simulink model "DA40_Flight_Model"  (R2023a)
settings: Solver=FixedStepAuto  StartTime=Start_Time  StopTime=End_Time  FixedStep=Time_Step  RelTol=1e-3
values from neighbouring files (symbols this model uses):
  BSFC_LUT = aircraft.BSFC_LUT    [NavigationProcessor.m]    (also in ReceiverPositions.m = obj.aircraft.BSFC_LUT; VectorTracking.m = load("DA40ENGINE.mat"))
  clkVar = formClkVariance(aircraft.clockType,1/aircraft.frequency)    [initializeSim.m]
  initP = blkdiag(diag([0.1 0.1 0.1]),diag([pi/90 pi/90 pi/90]),diag([1 1 1]),diag([pi/45 pi/45 pi/45]),clkVar)    [initializeSim.m]
  Q = blkdiag(diag(str2num(cell2mat(aircraft.noiseVariance))),clkVar)    [initializeSim.m]
  STGeometry = aircraft.STGeometry    [NavigationProcessor.m]    (also in ReceiverPositions.m = obj.aircraft.STGeometry; VectorTracking.m = load("DA40STGEOM.mat"))
  Vehicle = aircraft.Vehicle    [NavigationProcessor.m]    (also in ReceiverPositions.m = obj.aircraft.Vehicle; VectorTracking.m = load("DA40.mat"))
undefined symbols (not defined in the file or in its folder): day, initCN0, Initial_X, month, PowerFactor_LUT, Time_Step, unifrnd, variance, year
libraries: slpidlib x8, simulink_extras x3, aerolibwind2 x2, aerolibatmos2 x2, simulink x1
(part 1 of 2)
settings Model: Creator=izc0018  LastModifiedBy=nsm0014
settings OptimizationCC: ZeroExternalMemoryAtStartup=off  ZeroInternalMemoryAtStartup=off  InitFltsAndDblsToZero=on
settings DebuggingCC: AlgebraicLoopMsg=none  UnconnectedInputMsg=warning  UnconnectedOutputMsg=warning  UnconnectedLineMsg=warning
settings HardwareCC: ProdBitPerLong=64  ProdLargestAtomicFloat=None  ProdLongLongMode=on  ProdHWDeviceType=AMD->Athlon 64  TargetLongLongMode=on
settings ModelReferenceCC: EnableRefExpFcnMdlSchedulingChecks=on  ModelReferenceMinAlgLoopOccurrences=on
settings RTWCC: TargetLang=C++  GenerateGPUCode=CUDA  GPUMallocThreshold=400  GPUStackLimitPerThread=2048  GPUComputeCapability=8.6  DLArmComputeVersion=19.05
settings GRTTargetCC: TargetLangStandard=C++11 (ISO)  CodeInterfacePackaging=C++ class

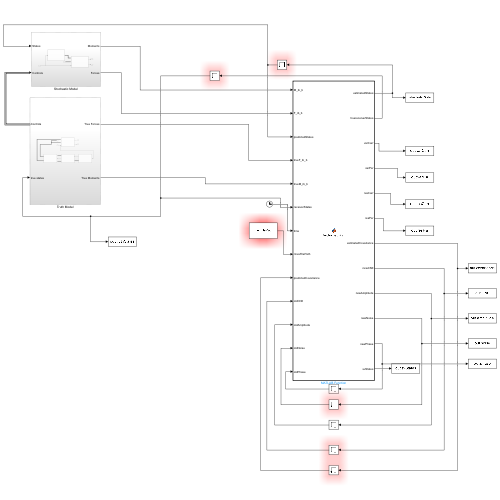
[thumbnail: Simulink's stored preview of the top-level diagram]
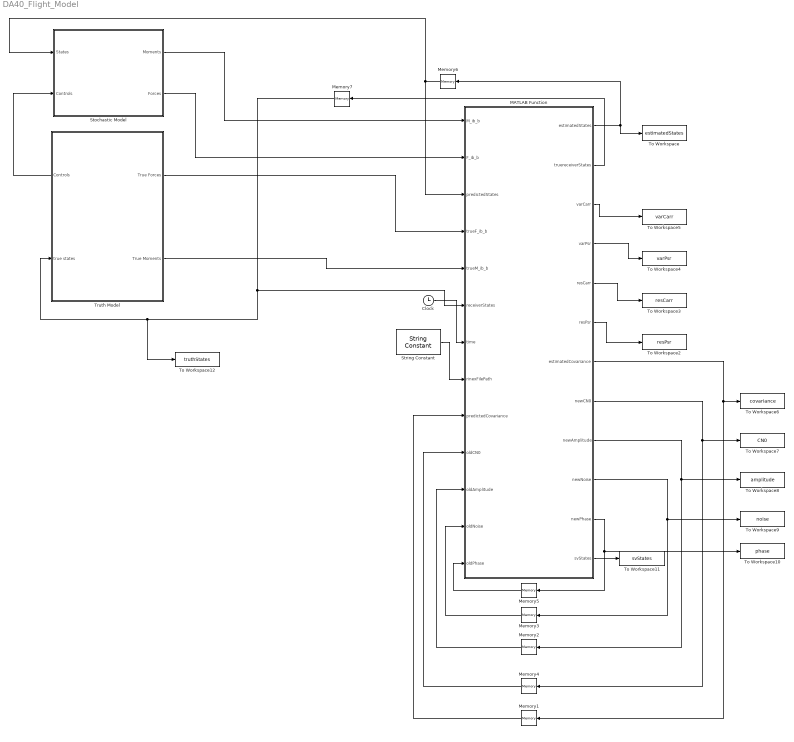
== system DA40_Flight_Model ==
  Clock : Clock
  MATLAB Function : MATLAB Function  TreatAsAtomicUnit=on
  Memory1 : Memory  InitialCondition=initP  InheritSampleTime=on  LinearizeMemory=on  LinearizeAsDelay=on
  Memory2 : Memory  InitialCondition=ones(1,31)  InheritSampleTime=on  LinearizeMemory=on  LinearizeAsDelay=on
  Memory3 : Memory  InitialCondition=1./(2*0.02*(initCN0))  InheritSampleTime=on  LinearizeMemory=on  LinearizeAsDelay=on
  Memory4 : Memory  InitialCondition=initCN0  InheritSampleTime=on  LinearizeMemory=on  LinearizeAsDelay=on
  Memory5 : Memory  InitialCondition=unifrnd(0,1,1,31)  InheritSampleTime=on  LinearizeMemory=on  LinearizeAsDelay=on
  Memory6 : Memory  InitialCondition=Initial_X  InheritSampleTime=on  LinearizeMemory=on  LinearizeAsDelay=on
  Memory7 : Memory  InitialCondition=Initial_X  InheritSampleTime=on  LinearizeMemory=on  LinearizeAsDelay=on
  Stochastic Model : Subsystem  SystemSampleTime=1/50
  String Constant : StringConstant  String=rinexFilePath
  To Workspace : ToWorkspace  VariableName=estimatedStates  SampleTime=-1
      settings: Save2DSignal=2-D array (concatenate along first dimension)
  To Workspace10 : ToWorkspace  VariableName=phase  SampleTime=-1
      settings: Save2DSignal=2-D array (concatenate along first dimension)
  To Workspace11 : ToWorkspace  VariableName=svStates  SampleTime=-1
  To Workspace12 : ToWorkspace  VariableName=truthStates  SampleTime=-1
      settings: Save2DSignal=2-D array (concatenate along first dimension)
  To Workspace2 : ToWorkspace  VariableName=resPsr  SampleTime=-1
      settings: Save2DSignal=2-D array (concatenate along first dimension)
  To Workspace3 : ToWorkspace  VariableName=resCarr  SampleTime=-1
      settings: Save2DSignal=2-D array (concatenate along first dimension)
  To Workspace4 : ToWorkspace  VariableName=varPsr  SampleTime=-1
      settings: Save2DSignal=2-D array (concatenate along first dimension)
  To Workspace5 : ToWorkspace  VariableName=varCarr  SampleTime=-1
      settings: Save2DSignal=2-D array (concatenate along first dimension)
  To Workspace6 : ToWorkspace  VariableName=covariance  SampleTime=-1
  To Workspace7 : ToWorkspace  VariableName=CN0  SampleTime=-1
      settings: Save2DSignal=2-D array (concatenate along first dimension)
  To Workspace8 : ToWorkspace  VariableName=amplitude  SampleTime=-1
      settings: Save2DSignal=2-D array (concatenate along first dimension)
  To Workspace9 : ToWorkspace  VariableName=noise  SampleTime=-1
      settings: Save2DSignal=2-D array (concatenate along first dimension)
  Truth Model : Subsystem  SystemSampleTime=1/50
      settings: PortSchema="{\"entries\":[{\"content\":{\"sides\":[{\"content\":{\"connectorIds\":[\"Out3\",\"In1\"]},\"type\":\"ConnectorPlacement.EquallySpacedRectSide\",\"uuid\":\"c5f3d2b3-4b9e-4074-adbc-162b6fd971ba\"},{\"content\":{\"connectorIds\":[\"Out1\",\"Out2\"],\"side\":\"RIGHT\"},\"type\":\"ConnectorPlacement.EquallySpacedRectSide\",\"uuid\":\"313b55c4-908f-4c38-afd9-9f2511d55f7a\"},{\"content\":{\"side\":\"TOP\"},\"type\":\"ConnectorPlacement.EquallySpacedRectSide\",\"uuid\":\"fab6a73b-2d20-4af2-8657-36bbff75e0c6\"}]},\"type\":\"ConnectorPlacement.EquallySpacedConnector\",\"uuid\":\"3c85a553-b056-4f11-83e7-abed49e05725\"}],\"packageUris\":[\"http://schema.mathworks.com/mf0/Connector/R2020b\"],\"version\":\"1.0\"}"
  wires:
  Clock/1 -> MATLAB Function/7(time)
  Memory3/1 -> MATLAB Function/12(oldNoise)
  MATLAB Function/8(newCN0) -> To Workspace7/1, Memory4/1
  MATLAB Function/4(varPsr) -> To Workspace4/1
  MATLAB Function/7(estimatedCovariance) -> To Workspace6/1, Memory1/1
  MATLAB Function/6(resPsr) -> To Workspace2/1
  Memory1/1 -> MATLAB Function/9(predictedCovariance)
  Memory5/1 -> MATLAB Function/13(oldPhase)
  MATLAB Function/9(newAmplitude) -> To Workspace8/1, Memory2/1
  MATLAB Function/5(resCarr) -> To Workspace3/1
  MATLAB Function/11(newPhase) -> Memory5/1, To Workspace10/1
  MATLAB Function/3(varCarr) -> To Workspace5/1
  Memory4/1 -> MATLAB Function/10(oldCN0)
  String Constant/1 -> MATLAB Function/8(rinexFilePath)
  Memory2/1 -> MATLAB Function/11(oldAmplitude)
  MATLAB Function/10(newNoise) -> To Workspace9/1, Memory3/1
  MATLAB Function/2(truereceiverStates) -> Memory7/1
  Memory6/1 -> MATLAB Function/3(predictedStates), Stochastic Model/1(States)
  MATLAB Function/1(estimatedStates) -> Memory6/1, To Workspace/1
  Truth Model/3(Controls) -> Stochastic Model/2(Controls)
  MATLAB Function/12(svStates) -> To Workspace11/1
  Truth Model/1(True Forces) -> MATLAB Function/4(trueF_ib_b)
  Truth Model/2(True Moments) -> MATLAB Function/5(trueM_ib_b)
  Memory7/1 -> To Workspace12/1, Truth Model/1(true states), MATLAB Function/6(receiverStates)
  Stochastic Model/1(Moments) -> MATLAB Function/1(M_ib_b)
  Stochastic Model/2(Forces) -> MATLAB Function/2(F_ib_b)

== system DA40_Flight_Model/Stochastic Model ==
  States : Inport
  Controls : Inport  Port=2
  Environment : Subsystem
  Navigation1 : Subsystem
  Moments : Outport
  Forces : Outport  Port=2
  wires:
  Environment/1(Atmos) -> Navigation1/1(Atmosphere)
  Navigation1/1(Forces) -> Forces/1
  Navigation1/2(Moments) -> Moments/1
  States/1 -> Environment/1(States), Navigation1/3(Estimated States)
  Controls/1 -> Navigation1/2(Controls)

== system DA40_Flight_Model/Truth Model ==
  true states : Inport
  Control : Subsystem
  Environment : Subsystem
  Guidance : Subsystem
  Navigation1 : Subsystem
  True Forces : Outport
  True Moments : Outport  Port=2
  Controls : Outport  Port=3
  wires:
  Control/1(Controls) -> Controls/1, Navigation1/2(Controls)
  Environment/2(Atmos) -> Guidance/2(Atmosphere)
  Guidance/1(Commands) -> Control/1(Commands)
  Environment/1(States Out) -> Guidance/1(States)
  Guidance/2(States Out) -> Control/2(States)
  Guidance/3(Atmos) -> Control/3(Atmos)
  Control/2(Atmosphere) -> Navigation1/1(Atmosphere)
  Navigation1/1(Forces) -> True Forces/1
  Navigation1/2(Moments) -> True Moments/1
  true states/1 -> Environment/1(States), Navigation1/3(true states)

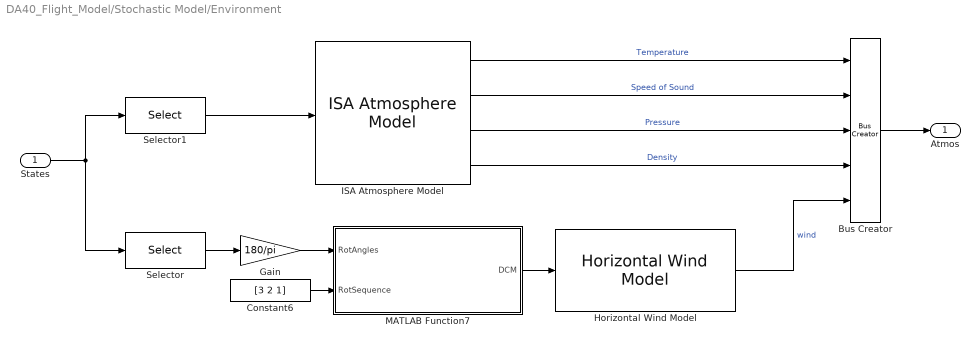
== system DA40_Flight_Model/Stochastic Model/Environment ==
  States : Inport
  Bus Creator : BusCreator  Inputs=5
  Constant6 : Constant  Value=[3 2 1]
  Gain : Gain  Gain=180/pi
  Horizontal Wind Model : aerolibwind2/Horizontal Wind Model  units=Metric (MKS)  Vw_source=Internal  Vwind=0  W_source=Internal  Wdeg=0
  ISA Atmosphere Model : aerolibatmos2/ISA Atmosphere Model  custom=off  g=9.80665  gamma=1.4  R=287.0531  L=0.0065  h_trop=11000  h_strat=20000  rho0=1.225  P0=101325  T0=288.15  h0=0
  MATLAB Function7 : MATLAB Function  TreatAsAtomicUnit=on
  Selector : Selector  InputPortWidth=14  IndexOptions=Index vector (dialog)  Indices=[10 11 12]  OutputSizes=1
  Selector1 : Selector  InputPortWidth=14  IndexOptions=Index vector (dialog)  Indices=[9]  OutputSizes=1
  Atmos : Outport
  wires:
  ISA Atmosphere Model/2 -> Bus Creator/2  "Speed of Sound"
  ISA Atmosphere Model/3 -> Bus Creator/3  "Pressure"
  Bus Creator/1 -> Atmos/1
  ISA Atmosphere Model/1 -> Bus Creator/1  "Temperature"
  Selector1/1 -> ISA Atmosphere Model/1
  ISA Atmosphere Model/4 -> Bus Creator/4  "Density"
  Gain/1 -> MATLAB Function7/1(RotAngles)
  MATLAB Function7/1(DCM) -> Horizontal Wind Model/1
  Constant6/1 -> MATLAB Function7/2(RotSequence)
  Selector/1 -> Gain/1
  States/1 -> Selector/1, Selector1/1
  Horizontal Wind Model/1 -> Bus Creator/5  "wind"

== system DA40_Flight_Model/Stochastic Model/Navigation1 ==
  Atmosphere : Inport
  Controls : Inport  Port=2
  Estimated States : Inport  Port=3
  Flight Mechanics and Systems Models : Subsystem
  Forces : Outport
  Moments : Outport  Port=2
  wires:
  Flight Mechanics and Systems Models/2(Mb) -> Moments/1
  Controls/1 -> Flight Mechanics and Systems Models/2(Control Commands)
  Atmosphere/1 -> Flight Mechanics and Systems Models/1(Atmosphere)
  Flight Mechanics and Systems Models/1(Fb) -> Forces/1
  Estimated States/1 -> Flight Mechanics and Systems Models/3(States)

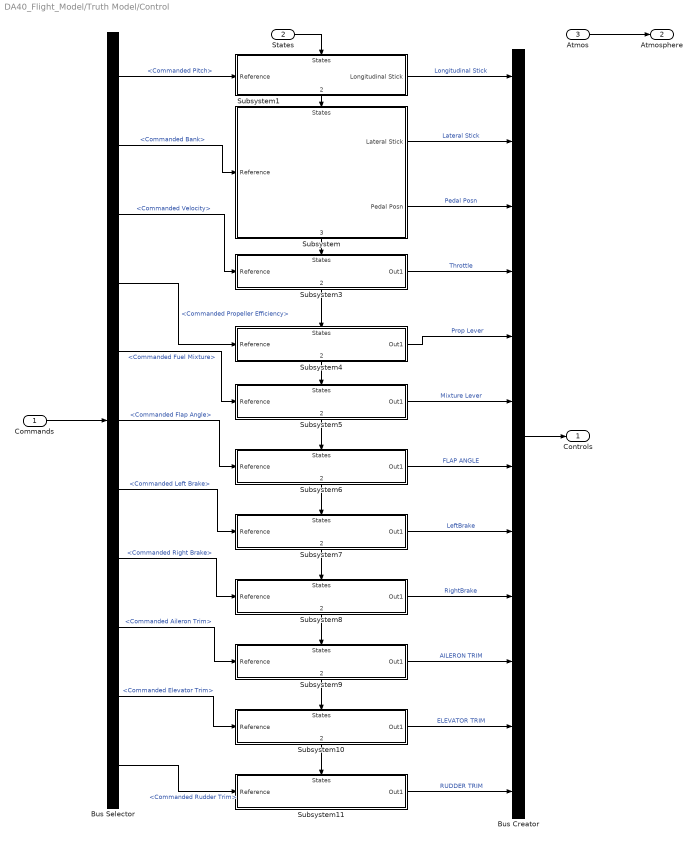
== system DA40_Flight_Model/Truth Model/Control ==
  Commands : Inport
  States : Inport  Port=2
  Atmos : Inport  Port=3
  Bus Creator : BusCreator  Inputs=12
  Bus Selector : BusSelector  OutputSignals=Commanded Pitch,Commanded Bank,Commanded Velocity,Commanded Propeller Efficiency,Commanded Fuel Mixture,Commanded Flap Angle,Commanded Left Brake,Commanded Right Brake,Commanded Aileron Trim,Commanded Elevator Trim,Commanded Rudder Trim
  Subsystem : Subsystem
      settings: PortSchema="{\"entries\":[{\"content\":{\"sides\":[{\"content\":{\"connectorIds\":[\"In1\"]},\"type\":\"ConnectorPlacement.EquallySpacedRectSide\",\"uuid\":\"5ea7349d-baf6-49c5-809d-4b912ce56d76\"},{\"content\":{\"connectorIds\":[\"Out1\",\"Out2\"],\"side\":\"RIGHT\"},\"type\":\"ConnectorPlacement.EquallySpacedRectSide\",\"uuid\":\"ab3ceec7-e245-42b0-9eb8-e3a68951e219\"},{\"content\":{\"connectorIds\":[\"In2\"],\"side\":\"TOP\"},\"type\":\"ConnectorPlacement.EquallySpacedRectSide\",\"uuid\":\"18178c43-0035-4aec-a3ba-011af3830f5c\"},{\"content\":{\"connectorIds\":[\"Out3\"],\"side\":\"BOTTOM\"},\"type\":\"ConnectorPlacement.EquallySpacedRectSide\",\"uuid\":\"88476787-2df8-4308-98f2-16231590cef9\"}]},\"type\":\"ConnectorPlacement.EquallySpacedConnector\",\"uuid\":\"0f7476f8-a4e6-4d2f-9698-249fd1b1cc90\"}],\"packageUris\":[\"http://schema.mathworks.com/mf0/Connector/R2020b\"],\"version\":\"1.0\"}"
  Subsystem1 : Subsystem
      settings: PortSchema="{\"entries\":[{\"content\":{\"sides\":[{\"content\":{\"connectorIds\":[\"In1\"]},\"type\":\"ConnectorPlacement.EquallySpacedRectSide\",\"uuid\":\"df1e81ab-d97f-43f0-8cd1-ba06c25288e8\"},{\"content\":{\"connectorIds\":[\"Out1\"],\"side\":\"RIGHT\"},\"type\":\"ConnectorPlacement.EquallySpacedRectSide\",\"uuid\":\"fe7f65be-8a13-42ab-8ffa-afe418a633fa\"},{\"content\":{\"connectorIds\":[\"In2\"],\"side\":\"TOP\"},\"type\":\"ConnectorPlacement.EquallySpacedRectSide\",\"uuid\":\"4762097a-1dfd-4646-aeb3-678774417eb9\"},{\"content\":{\"connectorIds\":[\"Out2\"],\"side\":\"BOTTOM\"},\"type\":\"ConnectorPlacement.EquallySpacedRectSide\",\"uuid\":\"338e28fc-4594-4f48-8379-f1c16de78061\"}]},\"type\":\"ConnectorPlacement.EquallySpacedConnector\",\"uuid\":\"e1e6a329-5243-44ef-b6a4-a2802fff17f2\"}],\"packageUris\":[\"http://schema.mathworks.com/mf0/Connector/R2020b\"],\"version\":\"1.0\"}"
  Subsystem10 : Subsystem
      settings: PortSchema="{\"entries\":[{\"content\":{\"sides\":[{\"content\":{\"connectorIds\":[\"In1\"]},\"type\":\"ConnectorPlacement.EquallySpacedRectSide\",\"uuid\":\"df1e81ab-d97f-43f0-8cd1-ba06c25288e8\"},{\"content\":{\"connectorIds\":[\"Out1\"],\"side\":\"RIGHT\"},\"type\":\"ConnectorPlacement.EquallySpacedRectSide\",\"uuid\":\"fe7f65be-8a13-42ab-8ffa-afe418a633fa\"},{\"content\":{\"connectorIds\":[\"In2\"],\"side\":\"TOP\"},\"type\":\"ConnectorPlacement.EquallySpacedRectSide\",\"uuid\":\"4762097a-1dfd-4646-aeb3-678774417eb9\"},{\"content\":{\"connectorIds\":[\"Out2\"],\"side\":\"BOTTOM\"},\"type\":\"ConnectorPlacement.EquallySpacedRectSide\",\"uuid\":\"ca232b1a-28ac-4e7a-b8a6-76103b2c6113\"}]},\"type\":\"ConnectorPlacement.EquallySpacedConnector\",\"uuid\":\"e1e6a329-5243-44ef-b6a4-a2802fff17f2\"}],\"packageUris\":[\"http://schema.mathworks.com/mf0/Connector/R2020b\"],\"version\":\"1.0\"}"
  Subsystem11 : Subsystem
      settings: PortSchema="{\"entries\":[{\"content\":{\"sides\":[{\"content\":{\"connectorIds\":[\"In1\"]},\"type\":\"ConnectorPlacement.EquallySpacedRectSide\",\"uuid\":\"df1e81ab-d97f-43f0-8cd1-ba06c25288e8\"},{\"content\":{\"connectorIds\":[\"Out1\"],\"side\":\"RIGHT\"},\"type\":\"ConnectorPlacement.EquallySpacedRectSide\",\"uuid\":\"fe7f65be-8a13-42ab-8ffa-afe418a633fa\"},{\"content\":{\"connectorIds\":[\"In2\"],\"side\":\"TOP\"},\"type\":\"ConnectorPlacement.EquallySpacedRectSide\",\"uuid\":\"4762097a-1dfd-4646-aeb3-678774417eb9\"}]},\"type\":\"ConnectorPlacement.EquallySpacedConnector\",\"uuid\":\"e1e6a329-5243-44ef-b6a4-a2802fff17f2\"}],\"packageUris\":[\"http://schema.mathworks.com/mf0/Connector/R2020b\"],\"version\":\"1.0\"}"
  Subsystem3 : Subsystem
      settings: PortSchema="{\"entries\":[{\"content\":{\"sides\":[{\"content\":{\"connectorIds\":[\"In1\"]},\"type\":\"ConnectorPlacement.EquallySpacedRectSide\",\"uuid\":\"df1e81ab-d97f-43f0-8cd1-ba06c25288e8\"},{\"content\":{\"connectorIds\":[\"Out1\"],\"side\":\"RIGHT\"},\"type\":\"ConnectorPlacement.EquallySpacedRectSide\",\"uuid\":\"fe7f65be-8a13-42ab-8ffa-afe418a633fa\"},{\"content\":{\"connectorIds\":[\"In2\"],\"side\":\"TOP\"},\"type\":\"ConnectorPlacement.EquallySpacedRectSide\",\"uuid\":\"4762097a-1dfd-4646-aeb3-678774417eb9\"},{\"content\":{\"connectorIds\":[\"Out2\"],\"side\":\"BOTTOM\"},\"type\":\"ConnectorPlacement.EquallySpacedRectSide\",\"uuid\":\"eb7acd08-7b98-4b28-a61a-3ca4385205ec\"}]},\"type\":\"ConnectorPlacement.EquallySpacedConnector\",\"uuid\":\"e1e6a329-5243-44ef-b6a4-a2802fff17f2\"}],\"packageUris\":[\"http://schema.mathworks.com/mf0/Connector/R2020b\"],\"version\":\"1.0\"}"
  Subsystem4 : Subsystem
      settings: PortSchema="{\"entries\":[{\"content\":{\"sides\":[{\"content\":{\"connectorIds\":[\"In1\"]},\"type\":\"ConnectorPlacement.EquallySpacedRectSide\",\"uuid\":\"df1e81ab-d97f-43f0-8cd1-ba06c25288e8\"},{\"content\":{\"connectorIds\":[\"Out1\"],\"side\":\"RIGHT\"},\"type\":\"ConnectorPlacement.EquallySpacedRectSide\",\"uuid\":\"fe7f65be-8a13-42ab-8ffa-afe418a633fa\"},{\"content\":{\"connectorIds\":[\"In2\"],\"side\":\"TOP\"},\"type\":\"ConnectorPlacement.EquallySpacedRectSide\",\"uuid\":\"4762097a-1dfd-4646-aeb3-678774417eb9\"},{\"content\":{\"connectorIds\":[\"Out2\"],\"side\":\"BOTTOM\"},\"type\":\"ConnectorPlacement.EquallySpacedRectSide\",\"uuid\":\"aca1bd27-9370-4c71-9435-0c269f9a438b\"}]},\"type\":\"ConnectorPlacement.EquallySpacedConnector\",\"uuid\":\"e1e6a329-5243-44ef-b6a4-a2802fff17f2\"}],\"packageUris\":[\"http://schema.mathworks.com/mf0/Connector/R2020b\"],\"version\":\"1.0\"}"
  Subsystem5 : Subsystem
      settings: PortSchema="{\"entries\":[{\"content\":{\"sides\":[{\"content\":{\"connectorIds\":[\"In1\"]},\"type\":\"ConnectorPlacement.EquallySpacedRectSide\",\"uuid\":\"df1e81ab-d97f-43f0-8cd1-ba06c25288e8\"},{\"content\":{\"connectorIds\":[\"Out1\"],\"side\":\"RIGHT\"},\"type\":\"ConnectorPlacement.EquallySpacedRectSide\",\"uuid\":\"fe7f65be-8a13-42ab-8ffa-afe418a633fa\"},{\"content\":{\"connectorIds\":[\"In2\"],\"side\":\"TOP\"},\"type\":\"ConnectorPlacement.EquallySpacedRectSide\",\"uuid\":\"4762097a-1dfd-4646-aeb3-678774417eb9\"},{\"content\":{\"connectorIds\":[\"Out2\"],\"side\":\"BOTTOM\"},\"type\":\"ConnectorPlacement.EquallySpacedRectSide\",\"uuid\":\"e3132084-5e8e-4693-9249-2c258902bcf1\"}]},\"type\":\"ConnectorPlacement.EquallySpacedConnector\",\"uuid\":\"e1e6a329-5243-44ef-b6a4-a2802fff17f2\"}],\"packageUris\":[\"http://schema.mathworks.com/mf0/Connector/R2020b\"],\"version\":\"1.0\"}"
  Subsystem6 : Subsystem
      settings: PortSchema="{\"entries\":[{\"content\":{\"sides\":[{\"content\":{\"connectorIds\":[\"In1\"]},\"type\":\"ConnectorPlacement.EquallySpacedRectSide\",\"uuid\":\"df1e81ab-d97f-43f0-8cd1-ba06c25288e8\"},{\"content\":{\"connectorIds\":[\"Out1\"],\"side\":\"RIGHT\"},\"type\":\"ConnectorPlacement.EquallySpacedRectSide\",\"uuid\":\"fe7f65be-8a13-42ab-8ffa-afe418a633fa\"},{\"content\":{\"connectorIds\":[\"In2\"],\"side\":\"TOP\"},\"type\":\"ConnectorPlacement.EquallySpacedRectSide\",\"uuid\":\"4762097a-1dfd-4646-aeb3-678774417eb9\"},{\"content\":{\"connectorIds\":[\"Out2\"],\"side\":\"BOTTOM\"},\"type\":\"ConnectorPlacement.EquallySpacedRectSide\",\"uuid\":\"44b8b4cf-3de4-40e9-9bc3-b7b2ed15b9c4\"}]},\"type\":\"ConnectorPlacement.EquallySpacedConnector\",\"uuid\":\"e1e6a329-5243-44ef-b6a4-a2802fff17f2\"}],\"packageUris\":[\"http://schema.mathworks.com/mf0/Connector/R2020b\"],\"version\":\"1.0\"}"
  Subsystem7 : Subsystem
      settings: PortSchema="{\"entries\":[{\"content\":{\"sides\":[{\"content\":{\"connectorIds\":[\"In1\"]},\"type\":\"ConnectorPlacement.EquallySpacedRectSide\",\"uuid\":\"df1e81ab-d97f-43f0-8cd1-ba06c25288e8\"},{\"content\":{\"connectorIds\":[\"Out1\"],\"side\":\"RIGHT\"},\"type\":\"ConnectorPlacement.EquallySpacedRectSide\",\"uuid\":\"fe7f65be-8a13-42ab-8ffa-afe418a633fa\"},{\"content\":{\"connectorIds\":[\"In2\"],\"side\":\"TOP\"},\"type\":\"ConnectorPlacement.EquallySpacedRectSide\",\"uuid\":\"4762097a-1dfd-4646-aeb3-678774417eb9\"},{\"content\":{\"connectorIds\":[\"Out2\"],\"side\":\"BOTTOM\"},\"type\":\"ConnectorPlacement.EquallySpacedRectSide\",\"uuid\":\"4aea28e3-05ae-492c-9523-17787d8052fd\"}]},\"type\":\"ConnectorPlacement.EquallySpacedConnector\",\"uuid\":\"e1e6a329-5243-44ef-b6a4-a2802fff17f2\"}],\"packageUris\":[\"http://schema.mathworks.com/mf0/Connector/R2020b\"],\"version\":\"1.0\"}"
  Subsystem8 : Subsystem
      settings: PortSchema="{\"entries\":[{\"content\":{\"sides\":[{\"content\":{\"connectorIds\":[\"In1\"]},\"type\":\"ConnectorPlacement.EquallySpacedRectSide\",\"uuid\":\"df1e81ab-d97f-43f0-8cd1-ba06c25288e8\"},{\"content\":{\"connectorIds\":[\"Out1\"],\"side\":\"RIGHT\"},\"type\":\"ConnectorPlacement.EquallySpacedRectSide\",\"uuid\":\"fe7f65be-8a13-42ab-8ffa-afe418a633fa\"},{\"content\":{\"connectorIds\":[\"In2\"],\"side\":\"TOP\"},\"type\":\"ConnectorPlacement.EquallySpacedRectSide\",\"uuid\":\"4762097a-1dfd-4646-aeb3-678774417eb9\"},{\"content\":{\"connectorIds\":[\"Out2\"],\"side\":\"BOTTOM\"},\"type\":\"ConnectorPlacement.EquallySpacedRectSide\",\"uuid\":\"60b425fe-182c-41c2-bc4c-aa97cb3d7ccf\"}]},\"type\":\"ConnectorPlacement.EquallySpacedConnector\",\"uuid\":\"e1e6a329-5243-44ef-b6a4-a2802fff17f2\"}],\"packageUris\":[\"http://schema.mathworks.com/mf0/Connector/R2020b\"],\"version\":\"1.0\"}"
  Subsystem9 : Subsystem
      settings: PortSchema="{\"entries\":[{\"content\":{\"sides\":[{\"content\":{\"connectorIds\":[\"In1\"]},\"type\":\"ConnectorPlacement.EquallySpacedRectSide\",\"uuid\":\"df1e81ab-d97f-43f0-8cd1-ba06c25288e8\"},{\"content\":{\"connectorIds\":[\"Out1\"],\"side\":\"RIGHT\"},\"type\":\"ConnectorPlacement.EquallySpacedRectSide\",\"uuid\":\"fe7f65be-8a13-42ab-8ffa-afe418a633fa\"},{\"content\":{\"connectorIds\":[\"In2\"],\"side\":\"TOP\"},\"type\":\"ConnectorPlacement.EquallySpacedRectSide\",\"uuid\":\"4762097a-1dfd-4646-aeb3-678774417eb9\"},{\"content\":{\"connectorIds\":[\"Out2\"],\"side\":\"BOTTOM\"},\"type\":\"ConnectorPlacement.EquallySpacedRectSide\",\"uuid\":\"88e2b07d-9cf7-412b-8368-04827ebf702b\"}]},\"type\":\"ConnectorPlacement.EquallySpacedConnector\",\"uuid\":\"e1e6a329-5243-44ef-b6a4-a2802fff17f2\"}],\"packageUris\":[\"http://schema.mathworks.com/mf0/Connector/R2020b\"],\"version\":\"1.0\"}"
  Controls : Outport
  Atmosphere : Outport  Port=2
  wires:
  Subsystem11/1(Out1) -> Bus Creator/12  "RUDDER TRIM"
  Subsystem9/1(Out1) -> Bus Creator/10  "AILERON TRIM"
  Subsystem1/1(Longitudinal Stick) -> Bus Creator/1  "Longitudinal Stick"
  Subsystem/1(Lateral Stick) -> Bus Creator/2  "Lateral Stick"
  Subsystem6/1(Out1) -> Bus Creator/7  "FLAP ANGLE"
  Subsystem5/1(Out1) -> Bus Creator/6  "Mixture Lever"
  Subsystem3/1(Out1) -> Bus Creator/4  "Throttle"
  Subsystem8/1(Out1) -> Bus Creator/9  "RightBrake"
  Subsystem/2(Pedal Posn) -> Bus Creator/3  "Pedal Posn"
  Subsystem4/1(Out1) -> Bus Creator/5  "Prop Lever"
  Subsystem7/1(Out1) -> Bus Creator/8  "LeftBrake"
  Subsystem10/1(Out1) -> Bus Creator/11  "ELEVATOR TRIM"
  Bus Creator/1 -> Controls/1
  Commands/1 -> Bus Selector/1
  Bus Selector/11 -> Subsystem11/1(Reference)  "<Commanded Rudder Trim>"
  Bus Selector/10 -> Subsystem10/1(Reference)  "<Commanded Elevator Trim>"
  Bus Selector/9 -> Subsystem9/1(Reference)  "<Commanded Aileron Trim>"
  Bus Selector/8 -> Subsystem8/1(Reference)  "<Commanded Right Brake>"
  Bus Selector/7 -> Subsystem7/1(Reference)  "<Commanded Left Brake>"
  Bus Selector/6 -> Subsystem6/1(Reference)  "<Commanded Flap Angle>"
  Bus Selector/5 -> Subsystem5/1(Reference)  "<Commanded Fuel Mixture>"
  Bus Selector/4 -> Subsystem4/1(Reference)  "<Commanded Propeller Efficiency>"
  Bus Selector/3 -> Subsystem3/1(Reference)  "<Commanded Velocity>"
  Bus Selector/1 -> Subsystem1/1(Reference)  "<Commanded Pitch>"
  Bus Selector/2 -> Subsystem/1(Reference)  "<Commanded Bank>"
  States/1 -> Subsystem1/2(States)
  Subsystem6/2(" ") -> Subsystem7/2(States)
  Subsystem9/2(" ") -> Subsystem10/2(States)
  Subsystem3/2(" ") -> Subsystem4/2(States)
  Subsystem/3(" ") -> Subsystem3/2(States)
  Subsystem1/2(" ") -> Subsystem/2(States)
  Subsystem7/2(" ") -> Subsystem8/2(States)
  Subsystem8/2(" ") -> Subsystem9/2(States)
  Subsystem5/2(" ") -> Subsystem6/2(States)
  Subsystem4/2(" ") -> Subsystem5/2(States)
  Subsystem10/2(" ") -> Subsystem11/2(States)
  Atmos/1 -> Atmosphere/1

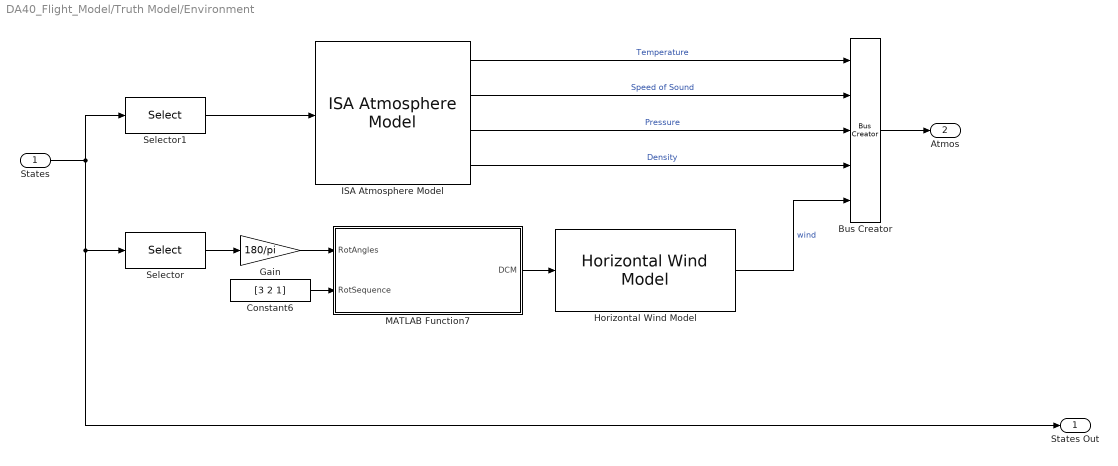
== system DA40_Flight_Model/Truth Model/Environment ==
  States : Inport
  Bus Creator : BusCreator  Inputs=5
  Constant6 : Constant  Value=[3 2 1]
  Gain : Gain  Gain=180/pi
  Horizontal Wind Model : aerolibwind2/Horizontal Wind Model  units=Metric (MKS)  Vw_source=Internal  Vwind=0  W_source=Internal  Wdeg=0
  ISA Atmosphere Model : aerolibatmos2/ISA Atmosphere Model  custom=off  g=9.80665  gamma=1.4  R=287.0531  L=0.0065  h_trop=11000  h_strat=20000  rho0=1.225  P0=101325  T0=288.15  h0=0
  MATLAB Function7 : MATLAB Function  TreatAsAtomicUnit=on
  Selector : Selector  InputPortWidth=14  IndexOptions=Index vector (dialog)  Indices=[10 11 12]  OutputSizes=1
  Selector1 : Selector  InputPortWidth=14  IndexOptions=Index vector (dialog)  Indices=[9]  OutputSizes=1
  States Out : Outport
  Atmos : Outport  Port=2
  wires:
  ISA Atmosphere Model/2 -> Bus Creator/2  "Speed of Sound"
  ISA Atmosphere Model/3 -> Bus Creator/3  "Pressure"
  Bus Creator/1 -> Atmos/1
  ISA Atmosphere Model/1 -> Bus Creator/1  "Temperature"
  Selector1/1 -> ISA Atmosphere Model/1
  ISA Atmosphere Model/4 -> Bus Creator/4  "Density"
  Gain/1 -> MATLAB Function7/1(RotAngles)
  MATLAB Function7/1(DCM) -> Horizontal Wind Model/1
  Constant6/1 -> MATLAB Function7/2(RotSequence)
  Selector/1 -> Gain/1
  States/1 -> Selector/1, States Out/1, Selector1/1
  Horizontal Wind Model/1 -> Bus Creator/5  "wind"

== system DA40_Flight_Model/Truth Model/Guidance ==
  States : Inport
  Atmosphere : Inport  Port=2
  Bus Creator : BusCreator  Inputs=11
  Radians to Degrees : simulink_extras/Transformations/Radians to Degrees
  Selector1 : Selector  InputPortWidth=14  IndexOptions=Index vector (dialog)  Indices=[12]  OutputSizes=1
  Subsystem : Subsystem
  Commands : Outport
  States Out : Outport  Port=2
  Atmos : Outport  Port=3
  wires:
  Bus Creator/1 -> Commands/1
  Subsystem/1(Bank) -> Bus Creator/1  "Commanded Bank"
  Subsystem/2(Pitch) -> Bus Creator/2  "Commanded Pitch"
  Subsystem/3(Velocity) -> Bus Creator/3  "Commanded Velocity"
  Subsystem/4(Propeller Efficiency) -> Bus Creator/4  "Commanded Propeller Efficiency"
  Subsystem/5(Fuel Efficiency) -> Bus Creator/5  "Commanded Fuel Mixture"
  Subsystem/6(Flap Angle) -> Bus Creator/6  "Commanded Flap Angle"
  Subsystem/7(Left Brake) -> Bus Creator/7  "Commanded Left Brake"
  Subsystem/8(Right Brake) -> Bus Creator/8  "Commanded Right Brake"
  Subsystem/9(Aileron trim) -> Bus Creator/9  "Commanded Aileron Trim"
  Subsystem/10(Elevator Trim) -> Bus Creator/10  "Commanded Elevator Trim"
  Subsystem/11(Rudder Trim) -> Bus Creator/11  "Commanded Rudder Trim"
  States/1 -> Selector1/1, States Out/1
  Atmosphere/1 -> Atmos/1
  Radians to Degrees/1 -> Subsystem/1(Heading)
  Selector1/1 -> Radians to Degrees/1

== system DA40_Flight_Model/Truth Model/Navigation1 ==
  Atmosphere : Inport
  Controls : Inport  Port=2
  true states : Inport  Port=3
  Flight Mechanics and Systems Models : Subsystem
  Forces : Outport
  Moments : Outport  Port=2
  wires:
  Flight Mechanics and Systems Models/2(Mb) -> Moments/1
  Controls/1 -> Flight Mechanics and Systems Models/2(Control Commands)
  Atmosphere/1 -> Flight Mechanics and Systems Models/1(Atmosphere)
  Flight Mechanics and Systems Models/1(Fb) -> Forces/1
  true states/1 -> Flight Mechanics and Systems Models/3(States)

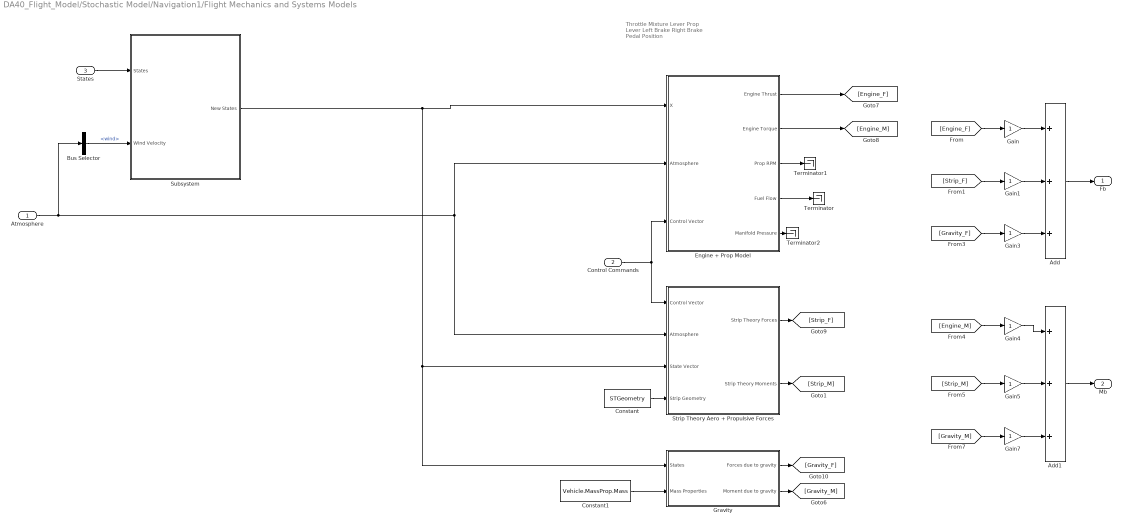
== system DA40_Flight_Model/Stochastic Model/Navigation1/Flight Mechanics and Systems Models ==
  note: Throttle
      | Mixture Lever
      | Prop Lever
      | Left Brake
      | Right Brake
      | Pedal Position
  Atmosphere : Inport
  Control Commands : Inport  Port=2
  States : Inport  Port=3
  Add : Sum  Inputs=+++
  Add1 : Sum  Inputs=+++
  Bus Selector : BusSelector  OutputSignals=wind
  Constant : Constant  Value=STGeometry
  Constant1 : Constant  Value=Vehicle.MassProp.Mass
  Engine + Prop Model : Subsystem
  Gain{,1,3..5,7} (6 alike) : Gain
  Gravity : Subsystem
  Strip Theory Aero + Propulsive Forces : Subsystem
  Subsystem : Subsystem
  Terminator : Terminator
  Terminator1 : Terminator
  Terminator2 : Terminator
  Fb : Outport
  Mb : Outport  Port=2
  wires:
  Constant1/1 -> Gravity/2(Mass Properties)
  Constant/1 -> Strip Theory Aero + Propulsive Forces/4(Strip Geometry)
  Engine + Prop Model/5(Manifold Pressure) -> Terminator2/1
  Engine + Prop Model/3(Prop RPM) -> Terminator1/1
  Add1/1 -> Mb/1
  Engine + Prop Model/2(Engine Torque) -> [Engine_M]
  Strip Theory Aero + Propulsive Forces/2(Strip Theory Moments) -> [Strip_M]
  Gravity/2(Moment due to gravity) -> [Gravity_M]
  Gravity/1(Forces due to gravity) -> [Gravity_F]
  Strip Theory Aero + Propulsive Forces/1(Strip Theory Forces) -> [Strip_F]
  Engine + Prop Model/1(Engine Thrust) -> [Engine_F]
  Add/1 -> Fb/1
  [Engine_F] -> Gain/1
  [Strip_F] -> Gain1/1
  [Gravity_F] -> Gain3/1
  [Engine_M] -> Gain4/1
  [Strip_M] -> Gain5/1
  [Gravity_M] -> Gain7/1
  Gain/1 -> Add/1
  Gain1/1 -> Add/2
  Gain3/1 -> Add/3
  Gain4/1 -> Add1/1
  Gain5/1 -> Add1/2
  Gain7/1 -> Add1/3
  Engine + Prop Model/4(Fuel Flow) -> Terminator/1
  Atmosphere/1 -> Bus Selector/1, Strip Theory Aero + Propulsive Forces/2(Atmosphere), Engine + Prop Model/2(Atmosphere)
  States/1 -> Subsystem/1(States)
  Control Commands/1 -> Strip Theory Aero + Propulsive Forces/1(Control Vector), Engine + Prop Model/3(Control Vector)
  Bus Selector/1 -> Subsystem/2(Wind Velocity)  "<wind>"
  Subsystem/1(New States) -> Gravity/1(States), Strip Theory Aero + Propulsive Forces/3(State Vector), Engine + Prop Model/1(X)

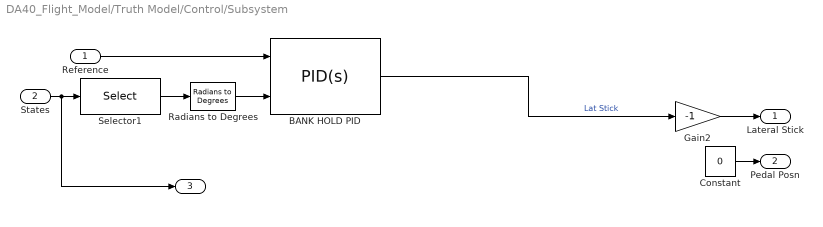
== system DA40_Flight_Model/Truth Model/Control/Subsystem ==
  Reference : Inport
  States : Inport  Port=2
  BANK HOLD PID : slpidlib/PID Controller (2DOF)  Controller=PID  Form=Parallel  TimeDomain=Continuous-time  UseExternalTs=off  SampleTime=-1  IntegratorMethod=Forward Euler  FilterMethod=Forward Euler  ControllerParametersSource=internal  P=0.107891692261891  I=0.133343747084316  UseKiTs=off  D=0.0171409705451499  N=25.8919437213056  UseFilter=on  b=0.548332573243903  c=0.00478750158934923  TunerSelectOption=Transfer Function Based (PID Tuner App)  InitialConditionSource=internal  InitialConditionForIntegrator=0  InitialConditionForFilter=0  DifferentiatorICPrevScaledInput=0  ExternalReset=none  TrackingMode=off  Kt=1  LimitOutput=on  SatLimitsSource=internal  UpperSaturationLimit=1  LowerSaturationLimit=-1  LinearizeAsGain=on  AntiWindupMode=clamping  Kb=1  LimitIntegrator=off  UpperIntegratorSaturationLimit=inf  LowerIntegratorSaturationLimit=-inf  POutMin=[]  POutMax=[]  IOutMin=[]  IOutMax=[]  DOutMin=[]  DOutMax=[]  NOutMin=[]  NOutMax=[]  bOutMin=[]  bOutMax=[]  cOutMin=[]  cOutMax=[]  SumOutMin=[]  SumOutMax=[]  SaturationOutMin=[]  SaturationOutMax=[]  PParamMin=[]  PParamMax=[]  IParamMin=[]  IParamMax=[]  DParamMin=[]  DParamMax=[]  NParamMin=[]  NParamMax=[]  bParamMin=[]  bParamMax=[]  cParamMin=[]  cParamMax=[]  KbParamMin=[]  KbParamMax=[]  KtParamMin=[]  KtParamMax=[]  KbOutMin=[]  KbOutMax=[]  KtOutMin=[]  KtOutMax=[]  IntegratorOutMin=[]  IntegratorOutMax=[]  FilterOutMin=[]  FilterOutMax=[]  SumI1OutMin=[]  SumI1OutMax=[]  SumI2OutMin=[]  SumI2OutMax=[]  SumI3OutMin=[]  SumI3OutMax=[]  SumI4OutMin=[]  SumI4OutMax=[]  SumDOutMin=[]  SumDOutMax=[]  Sum1OutMin=[]  Sum1OutMax=[]  Sum2OutMin=[]  Sum2OutMax=[]  Sum3OutMin=[]  Sum3OutMax=[]  DifferentiatorOutMin=[]  DifferentiatorOutMax=[]  FilterDiffOutCoefMin=[]  FilterDiffOutCoefMax=[]  ReciprocalOutMin=[]  ReciprocalOutMax=[]  SumDenOutMin=[]  SumDenOutMax=[]  SumNumOutMin=[]  SumNumOutMax=[]  DivideOutMin=[]  DivideOutMax=[]  UdiffTsProdOutMin=[]  UdiffTsProdOutMax=[]  NTsProdOutMin=[]  NTsProdOutMax=[]  UintegralTsProdOutMin=[]  UintegralTsProdOutMax=[]  UngainTsProdOutMin=[]  UngainTsProdOutMax=[]  ClampingZeroOutDataTypeStr=Inherit: Inherit via back propagation  ClampingZeroOutMin=[]  ClampingZeroOutMax=[]  FilterDenConstantOutDataTypeStr=Inherit: Inherit via back propagation  FilterDenConstantOutMin=[]  FilterDenConstantOutMax=[]  PCopyOutDataTypeStr=Inherit: Inherit via back propagation  PCopyOutMin=[]  PCopyOutMax=[]  NCopyOutDataTypeStr=Inherit: Inherit via back propagation  NCopyOutMin=[]  NCopyOutMax=[]  IntegratorContinuousStateAttributes=''  IntegratorStateMustResolveToSignalObject=off  IntegratorRTWStateStorageClass=Auto  FilterContinuousStateAttributes=''  FilterStateMustResolveToSignalObject=off  FilterRTWStateStorageClass=Auto  ParallelPVariant=InternalParameters  IdealPVariant=Disabled  IVariant=InternalParameters  DVariant=InternalParameters  bVariant=InternalParameters  cVariant=InternalParameters  IntegratorVariant=Continuous  SatVariant=Enabled  AWVariant=ContClampingParallel  PCopyVariant=Disabled  TRVariant=Disabled  FdbkBlocksVariant=Forward  IdealPFdbkVariant=Disabled  SatFdbkVariant=Disabled  DerivativeFilterVariant=ContFilter  NVariant=InternalParameters  NCopyVariant=Disabled  FilterICVariant=InternalICsFilter  IntegratorICVariant=InternalICs  ExternalResetVariant=Disabled  TRSumVariant=Passthrough  SumFdbkVariant=Disabled  SumVariant=Sum_PID  TsampFilterVariant=InternalTs  TsampNgainVariant=Passthrough  TsampIntegralVariant=Disabled_SignalSpec  ExternalSaturationOutDataTypeStr=Inherit: Same as second input
  Constant : Constant  Value=0
  Gain2 : Gain  Gain=-1
  Radians to Degrees : simulink_extras/Transformations/Radians to Degrees
  Selector1 : Selector  InputPortWidth=14  IndexOptions=Index vector (dialog)  Indices=[10]  OutputSizes=1
  Lateral Stick : Outport
  Pedal Posn : Outport  Port=2
  " " : Outport  Port=3
  wires:
  Gain2/1 -> Lateral Stick/1
  Radians to Degrees/1 -> BANK HOLD PID/2
  States/1 -> Selector1/1, " "/1
  Selector1/1 -> Radians to Degrees/1
  Reference/1 -> BANK HOLD PID/1
  Constant/1 -> Pedal Posn/1
  BANK HOLD PID/1 -> Gain2/1  "Lat Stick"

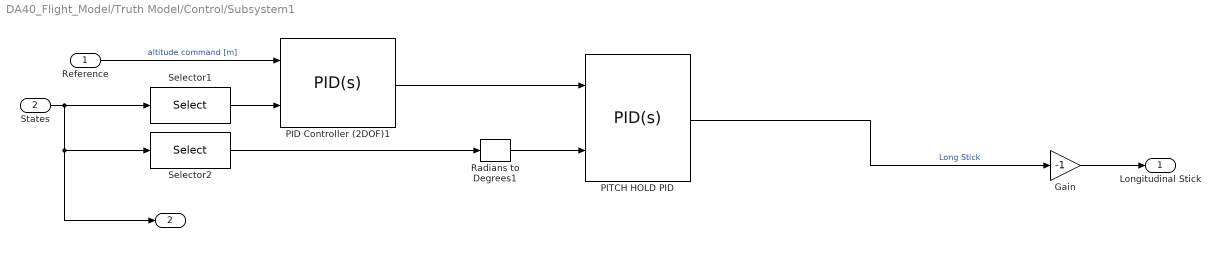
== system DA40_Flight_Model/Truth Model/Control/Subsystem1 ==
  Reference : Inport
  States : Inport  Port=2
  Gain : Gain  Gain=-1
  PID Controller (2DOF)1 : slpidlib/PID Controller (2DOF)  Controller=PID  Form=Parallel  TimeDomain=Continuous-time  UseExternalTs=off  SampleTime=-1  IntegratorMethod=Forward Euler  FilterMethod=Forward Euler  ControllerParametersSource=internal  P=0.392178102036374  I=0.0013184227867295  UseKiTs=off  D=-0.0973934682361479  N=4.02673925817559  UseFilter=on  b=1  c=1  TunerSelectOption=Transfer Function Based (PID Tuner App)  InitialConditionSource=internal  InitialConditionForIntegrator=0  InitialConditionForFilter=0  DifferentiatorICPrevScaledInput=0  ExternalReset=none  TrackingMode=off  Kt=1  LimitOutput=on  SatLimitsSource=internal  UpperSaturationLimit=15  LowerSaturationLimit=-15  LinearizeAsGain=on  AntiWindupMode=clamping  Kb=1  LimitIntegrator=off  UpperIntegratorSaturationLimit=inf  LowerIntegratorSaturationLimit=-inf  POutMin=[]  POutMax=[]  IOutMin=[]  IOutMax=[]  DOutMin=[]  DOutMax=[]  NOutMin=[]  NOutMax=[]  bOutMin=[]  bOutMax=[]  cOutMin=[]  cOutMax=[]  SumOutMin=[]  SumOutMax=[]  SaturationOutMin=[]  SaturationOutMax=[]  PParamMin=[]  PParamMax=[]  IParamMin=[]  IParamMax=[]  DParamMin=[]  DParamMax=[]  NParamMin=[]  NParamMax=[]  bParamMin=[]  bParamMax=[]  cParamMin=[]  cParamMax=[]  KbParamMin=[]  KbParamMax=[]  KtParamMin=[]  KtParamMax=[]  KbOutMin=[]  KbOutMax=[]  KtOutMin=[]  KtOutMax=[]  IntegratorOutMin=[]  IntegratorOutMax=[]  FilterOutMin=[]  FilterOutMax=[]  SumI1OutMin=[]  SumI1OutMax=[]  SumI2OutMin=[]  SumI2OutMax=[]  SumI3OutMin=[]  SumI3OutMax=[]  SumI4OutMin=[]  SumI4OutMax=[]  SumDOutMin=[]  SumDOutMax=[]  Sum1OutMin=[]  Sum1OutMax=[]  Sum2OutMin=[]  Sum2OutMax=[]  Sum3OutMin=[]  Sum3OutMax=[]  DifferentiatorOutMin=[]  DifferentiatorOutMax=[]  FilterDiffOutCoefMin=[]  FilterDiffOutCoefMax=[]  ReciprocalOutMin=[]  ReciprocalOutMax=[]  SumDenOutMin=[]  SumDenOutMax=[]  SumNumOutMin=[]  SumNumOutMax=[]  DivideOutMin=[]  DivideOutMax=[]  UdiffTsProdOutMin=[]  UdiffTsProdOutMax=[]  NTsProdOutMin=[]  NTsProdOutMax=[]  UintegralTsProdOutMin=[]  UintegralTsProdOutMax=[]  UngainTsProdOutMin=[]  UngainTsProdOutMax=[]  ClampingZeroOutDataTypeStr=Inherit: Inherit via back propagation  ClampingZeroOutMin=[]  ClampingZeroOutMax=[]  FilterDenConstantOutDataTypeStr=Inherit: Inherit via back propagation  FilterDenConstantOutMin=[]  FilterDenConstantOutMax=[]  PCopyOutDataTypeStr=Inherit: Inherit via back propagation  PCopyOutMin=[]  PCopyOutMax=[]  NCopyOutDataTypeStr=Inherit: Inherit via back propagation  NCopyOutMin=[]  NCopyOutMax=[]  IntegratorContinuousStateAttributes=''  IntegratorStateMustResolveToSignalObject=off  IntegratorRTWStateStorageClass=Auto  FilterContinuousStateAttributes=''  FilterStateMustResolveToSignalObject=off  FilterRTWStateStorageClass=Auto  ParallelPVariant=InternalParameters  IdealPVariant=Disabled  IVariant=InternalParameters  DVariant=InternalParameters  bVariant=InternalParameters  cVariant=InternalParameters  IntegratorVariant=Continuous  SatVariant=Enabled  AWVariant=ContClampingParallel  PCopyVariant=Disabled  TRVariant=Disabled  FdbkBlocksVariant=Forward  IdealPFdbkVariant=Disabled  SatFdbkVariant=Disabled  DerivativeFilterVariant=ContFilter  NVariant=InternalParameters  NCopyVariant=Disabled  FilterICVariant=InternalICsFilter  IntegratorICVariant=InternalICs  ExternalResetVariant=Disabled  TRSumVariant=Passthrough  SumFdbkVariant=Disabled  SumVariant=Sum_PID  TsampFilterVariant=InternalTs  TsampNgainVariant=Passthrough  TsampIntegralVariant=Disabled_SignalSpec  ExternalSaturationOutDataTypeStr=Inherit: Same as second input
  PITCH HOLD PID : slpidlib/PID Controller (2DOF)  Controller=PID  Form=Parallel  TimeDomain=Continuous-time  UseExternalTs=off  SampleTime=-1  IntegratorMethod=Forward Euler  FilterMethod=Forward Euler  ControllerParametersSource=internal  P=0.06  I=0.01  UseKiTs=off  D=0.02  N=100  UseFilter=on  b=1  c=0  TunerSelectOption=Transfer Function Based (PID Tuner App)  InitialConditionSource=internal  InitialConditionForIntegrator=0  InitialConditionForFilter=0  DifferentiatorICPrevScaledInput=0  ExternalReset=none  TrackingMode=off  Kt=1  LimitOutput=on  SatLimitsSource=internal  UpperSaturationLimit=1  LowerSaturationLimit=-1  LinearizeAsGain=on  AntiWindupMode=clamping  Kb=1  LimitIntegrator=off  UpperIntegratorSaturationLimit=inf  LowerIntegratorSaturationLimit=-inf  POutMin=[]  POutMax=[]  IOutMin=[]  IOutMax=[]  DOutMin=[]  DOutMax=[]  NOutMin=[]  NOutMax=[]  bOutMin=[]  bOutMax=[]  cOutMin=[]  cOutMax=[]  SumOutMin=[]  SumOutMax=[]  SaturationOutMin=[]  SaturationOutMax=[]  PParamMin=[]  PParamMax=[]  IParamMin=[]  IParamMax=[]  DParamMin=[]  DParamMax=[]  NParamMin=[]  NParamMax=[]  bParamMin=[]  bParamMax=[]  cParamMin=[]  cParamMax=[]  KbParamMin=[]  KbParamMax=[]  KtParamMin=[]  KtParamMax=[]  KbOutMin=[]  KbOutMax=[]  KtOutMin=[]  KtOutMax=[]  IntegratorOutMin=[]  IntegratorOutMax=[]  FilterOutMin=[]  FilterOutMax=[]  SumI1OutMin=[]  SumI1OutMax=[]  SumI2OutMin=[]  SumI2OutMax=[]  SumI3OutMin=[]  SumI3OutMax=[]  SumI4OutMin=[]  SumI4OutMax=[]  SumDOutMin=[]  SumDOutMax=[]  Sum1OutMin=[]  Sum1OutMax=[]  Sum2OutMin=[]  Sum2OutMax=[]  Sum3OutMin=[]  Sum3OutMax=[]  DifferentiatorOutMin=[]  DifferentiatorOutMax=[]  FilterDiffOutCoefMin=[]  FilterDiffOutCoefMax=[]  ReciprocalOutMin=[]  ReciprocalOutMax=[]  SumDenOutMin=[]  SumDenOutMax=[]  SumNumOutMin=[]  SumNumOutMax=[]  DivideOutMin=[]  DivideOutMax=[]  UdiffTsProdOutMin=[]  UdiffTsProdOutMax=[]  NTsProdOutMin=[]  NTsProdOutMax=[]  UintegralTsProdOutMin=[]  UintegralTsProdOutMax=[]  UngainTsProdOutMin=[]  UngainTsProdOutMax=[]  ClampingZeroOutDataTypeStr=Inherit: Inherit via back propagation  ClampingZeroOutMin=[]  ClampingZeroOutMax=[]  FilterDenConstantOutDataTypeStr=Inherit: Inherit via back propagation  FilterDenConstantOutMin=[]  FilterDenConstantOutMax=[]  PCopyOutDataTypeStr=Inherit: Inherit via back propagation  PCopyOutMin=[]  PCopyOutMax=[]  NCopyOutDataTypeStr=Inherit: Inherit via back propagation  NCopyOutMin=[]  NCopyOutMax=[]  IntegratorContinuousStateAttributes=''  IntegratorStateMustResolveToSignalObject=off  IntegratorRTWStateStorageClass=Auto  FilterContinuousStateAttributes=''  FilterStateMustResolveToSignalObject=off  FilterRTWStateStorageClass=Auto  ParallelPVariant=InternalParameters  IdealPVariant=Disabled  IVariant=InternalParameters  DVariant=InternalParameters  bVariant=InternalParameters  cVariant=InternalParameters  IntegratorVariant=Continuous  SatVariant=Enabled  AWVariant=ContClampingParallel  PCopyVariant=Disabled  TRVariant=Disabled  FdbkBlocksVariant=Forward  IdealPFdbkVariant=Disabled  SatFdbkVariant=Disabled  DerivativeFilterVariant=ContFilter  NVariant=InternalParameters  NCopyVariant=Disabled  FilterICVariant=InternalICsFilter  IntegratorICVariant=InternalICs  ExternalResetVariant=Disabled  TRSumVariant=Passthrough  SumFdbkVariant=Disabled  SumVariant=Sum_PID  TsampFilterVariant=InternalTs  TsampNgainVariant=Passthrough  TsampIntegralVariant=Disabled_SignalSpec  ExternalSaturationOutDataTypeStr=Inherit: Same as second input
  Radians to Degrees1 : simulink_extras/Transformations/Radians to Degrees
  Selector1 : Selector  InputPortWidth=14  IndexOptions=Index vector (dialog)  Indices=[9]  OutputSizes=1
  Selector2 : Selector  InputPortWidth=14  IndexOptions=Index vector (dialog)  Indices=[11]  OutputSizes=1
  Longitudinal Stick : Outport
  " " : Outport  Port=2
  wires:
  PID Controller (2DOF)1/1 -> PITCH HOLD PID/1
  Reference/1 -> PID Controller (2DOF)1/1  "altitude command [m]"
  Radians to Degrees1/1 -> PITCH HOLD PID/2
  States/1 -> Selector1/1, Selector2/1, " "/1
  Gain/1 -> Longitudinal Stick/1
  Selector1/1 -> PID Controller (2DOF)1/2
  Selector2/1 -> Radians to Degrees1/1
  PITCH HOLD PID/1 -> Gain/1  "Long Stick"

== system DA40_Flight_Model/Truth Model/Control/Subsystem10 ==
  Reference : Inport
  States : Inport  Port=2
  Out1 : Outport
  " " : Outport  Port=2
  wires:
  Reference/1 -> Out1/1
  States/1 -> " "/1

== system DA40_Flight_Model/Truth Model/Control/Subsystem11 ==
  Reference : Inport
  States : Inport  Port=2
  Terminator : Terminator
  Out1 : Outport
  wires:
  Reference/1 -> Out1/1
  States/1 -> Terminator/1

== system DA40_Flight_Model/Truth Model/Control/Subsystem3 ==
  Reference : Inport
  States : Inport  Port=2
  MATLAB Function : MATLAB Function  TreatAsAtomicUnit=on
  PID Controller (2DOF) : slpidlib/PID Controller (2DOF)  Controller=PID  Form=Parallel  TimeDomain=Continuous-time  UseExternalTs=off  SampleTime=-1  IntegratorMethod=Forward Euler  FilterMethod=Forward Euler  ControllerParametersSource=internal  P=0.497904922106352  I=0.0979272469433752  UseKiTs=off  D=-0.183968459268293  N=2.70646894628946  UseFilter=on  b=0.574546090887085  c=0.574546090887085  TunerSelectOption=Transfer Function Based (PID Tuner App)  InitialConditionSource=internal  InitialConditionForIntegrator=0  InitialConditionForFilter=0  DifferentiatorICPrevScaledInput=0  ExternalReset=none  TrackingMode=off  Kt=1  LimitOutput=on  SatLimitsSource=internal  UpperSaturationLimit=1  LowerSaturationLimit=0  LinearizeAsGain=on  AntiWindupMode=none  Kb=1  LimitIntegrator=off  UpperIntegratorSaturationLimit=inf  LowerIntegratorSaturationLimit=-inf  POutMin=[]  POutMax=[]  IOutMin=[]  IOutMax=[]  DOutMin=[]  DOutMax=[]  NOutMin=[]  NOutMax=[]  bOutMin=[]  bOutMax=[]  cOutMin=[]  cOutMax=[]  SumOutMin=[]  SumOutMax=[]  SaturationOutMin=[]  SaturationOutMax=[]  PParamMin=[]  PParamMax=[]  IParamMin=[]  IParamMax=[]  DParamMin=[]  DParamMax=[]  NParamMin=[]  NParamMax=[]  bParamMin=[]  bParamMax=[]  cParamMin=[]  cParamMax=[]  KbParamMin=[]  KbParamMax=[]  KtParamMin=[]  KtParamMax=[]  KbOutMin=[]  KbOutMax=[]  KtOutMin=[]  KtOutMax=[]  IntegratorOutMin=[]  IntegratorOutMax=[]  FilterOutMin=[]  FilterOutMax=[]  SumI1OutMin=[]  SumI1OutMax=[]  SumI2OutMin=[]  SumI2OutMax=[]  SumI3OutMin=[]  SumI3OutMax=[]  SumI4OutMin=[]  SumI4OutMax=[]  SumDOutMin=[]  SumDOutMax=[]  Sum1OutMin=[]  Sum1OutMax=[]  Sum2OutMin=[]  Sum2OutMax=[]  Sum3OutMin=[]  Sum3OutMax=[]  DifferentiatorOutMin=[]  DifferentiatorOutMax=[]  FilterDiffOutCoefMin=[]  FilterDiffOutCoefMax=[]  ReciprocalOutMin=[]  ReciprocalOutMax=[]  SumDenOutMin=[]  SumDenOutMax=[]  SumNumOutMin=[]  SumNumOutMax=[]  DivideOutMin=[]  DivideOutMax=[]  UdiffTsProdOutMin=[]  UdiffTsProdOutMax=[]  NTsProdOutMin=[]  NTsProdOutMax=[]  UintegralTsProdOutMin=[]  UintegralTsProdOutMax=[]  UngainTsProdOutMin=[]  UngainTsProdOutMax=[]  ClampingZeroOutDataTypeStr=Inherit: Inherit via back propagation  ClampingZeroOutMin=[]  ClampingZeroOutMax=[]  FilterDenConstantOutDataTypeStr=Inherit: Inherit via back propagation  FilterDenConstantOutMin=[]  FilterDenConstantOutMax=[]  PCopyOutDataTypeStr=Inherit: Inherit via back propagation  PCopyOutMin=[]  PCopyOutMax=[]  NCopyOutDataTypeStr=Inherit: Inherit via back propagation  NCopyOutMin=[]  NCopyOutMax=[]  IntegratorContinuousStateAttributes=''  IntegratorStateMustResolveToSignalObject=off  IntegratorRTWStateStorageClass=Auto  FilterContinuousStateAttributes=''  FilterStateMustResolveToSignalObject=off  FilterRTWStateStorageClass=Auto  ParallelPVariant=InternalParameters  IdealPVariant=Disabled  IVariant=InternalParameters  DVariant=InternalParameters  bVariant=InternalParameters  cVariant=InternalParameters  IntegratorVariant=Continuous  SatVariant=Enabled  AWVariant=Passthrough  PCopyVariant=Disabled  TRVariant=Disabled  FdbkBlocksVariant=Forward  IdealPFdbkVariant=Disabled  SatFdbkVariant=Disabled  DerivativeFilterVariant=ContFilter  NVariant=InternalParameters  NCopyVariant=Disabled  FilterICVariant=InternalICsFilter  IntegratorICVariant=InternalICs  ExternalResetVariant=Disabled  TRSumVariant=Passthrough  SumFdbkVariant=Disabled  SumVariant=Sum_PID  TsampFilterVariant=InternalTs  TsampNgainVariant=Passthrough  TsampIntegralVariant=Disabled_SignalSpec  ExternalSaturationOutDataTypeStr=Inherit: Same as second input
  Out1 : Outport
  " " : Outport  Port=2
  wires:
  PID Controller (2DOF)/1 -> Out1/1
  States/1 -> " "/1, MATLAB Function/1(X)
  MATLAB Function/1(Aircraft_Airspeed) -> PID Controller (2DOF)/2
  Reference/1 -> PID Controller (2DOF)/1

== system DA40_Flight_Model/Truth Model/Control/Subsystem4 ==
  Reference : Inport
  States : Inport  Port=2
  Display : Display
  Display1 : Display
  Display2 : Display
  PID Controller (2DOF) : slpidlib/PID Controller (2DOF)  Controller=PID  Form=Parallel  TimeDomain=Continuous-time  UseExternalTs=off  SampleTime=-1  IntegratorMethod=Forward Euler  FilterMethod=Forward Euler  ControllerParametersSource=internal  P=0  I=1  UseKiTs=off  D=0  N=100  UseFilter=on  b=1  c=1  TunerSelectOption=Transfer Function Based (PID Tuner App)  InitialConditionSource=internal  InitialConditionForIntegrator=0  InitialConditionForFilter=0  DifferentiatorICPrevScaledInput=0  ExternalReset=none  TrackingMode=off  Kt=1  LimitOutput=on  SatLimitsSource=internal  UpperSaturationLimit=1  LowerSaturationLimit=0  LinearizeAsGain=on  AntiWindupMode=none  Kb=1  LimitIntegrator=off  UpperIntegratorSaturationLimit=inf  LowerIntegratorSaturationLimit=-inf  POutMin=[]  POutMax=[]  IOutMin=[]  IOutMax=[]  DOutMin=[]  DOutMax=[]  NOutMin=[]  NOutMax=[]  bOutMin=[]  bOutMax=[]  cOutMin=[]  cOutMax=[]  SumOutMin=[]  SumOutMax=[]  SaturationOutMin=[]  SaturationOutMax=[]  PParamMin=[]  PParamMax=[]  IParamMin=[]  IParamMax=[]  DParamMin=[]  DParamMax=[]  NParamMin=[]  NParamMax=[]  bParamMin=[]  bParamMax=[]  cParamMin=[]  cParamMax=[]  KbParamMin=[]  KbParamMax=[]  KtParamMin=[]  KtParamMax=[]  KbOutMin=[]  KbOutMax=[]  KtOutMin=[]  KtOutMax=[]  IntegratorOutMin=[]  IntegratorOutMax=[]  FilterOutMin=[]  FilterOutMax=[]  SumI1OutMin=[]  SumI1OutMax=[]  SumI2OutMin=[]  SumI2OutMax=[]  SumI3OutMin=[]  SumI3OutMax=[]  SumI4OutMin=[]  SumI4OutMax=[]  SumDOutMin=[]  SumDOutMax=[]  Sum1OutMin=[]  Sum1OutMax=[]  Sum2OutMin=[]  Sum2OutMax=[]  Sum3OutMin=[]  Sum3OutMax=[]  DifferentiatorOutMin=[]  DifferentiatorOutMax=[]  FilterDiffOutCoefMin=[]  FilterDiffOutCoefMax=[]  ReciprocalOutMin=[]  ReciprocalOutMax=[]  SumDenOutMin=[]  SumDenOutMax=[]  SumNumOutMin=[]  SumNumOutMax=[]  DivideOutMin=[]  DivideOutMax=[]  UdiffTsProdOutMin=[]  UdiffTsProdOutMax=[]  NTsProdOutMin=[]  NTsProdOutMax=[]  UintegralTsProdOutMin=[]  UintegralTsProdOutMax=[]  UngainTsProdOutMin=[]  UngainTsProdOutMax=[]  ClampingZeroOutDataTypeStr=Inherit: Inherit via back propagation  ClampingZeroOutMin=[]  ClampingZeroOutMax=[]  FilterDenConstantOutDataTypeStr=Inherit: Inherit via back propagation  FilterDenConstantOutMin=[]  FilterDenConstantOutMax=[]  PCopyOutDataTypeStr=Inherit: Inherit via back propagation  PCopyOutMin=[]  PCopyOutMax=[]  NCopyOutDataTypeStr=Inherit: Inherit via back propagation  NCopyOutMin=[]  NCopyOutMax=[]  IntegratorContinuousStateAttributes=''  IntegratorStateMustResolveToSignalObject=off  IntegratorRTWStateStorageClass=Auto  FilterContinuousStateAttributes=''  FilterStateMustResolveToSignalObject=off  FilterRTWStateStorageClass=Auto  ParallelPVariant=InternalParameters  IdealPVariant=Disabled  IVariant=InternalParameters  DVariant=InternalParameters  bVariant=InternalParameters  cVariant=InternalParameters  IntegratorVariant=Continuous  SatVariant=Enabled  AWVariant=Passthrough  PCopyVariant=Disabled  TRVariant=Disabled  FdbkBlocksVariant=Forward  IdealPFdbkVariant=Disabled  SatFdbkVariant=Disabled  DerivativeFilterVariant=ContFilter  NVariant=InternalParameters  NCopyVariant=Disabled  FilterICVariant=InternalICsFilter  IntegratorICVariant=InternalICs  ExternalResetVariant=Disabled  TRSumVariant=Passthrough  SumFdbkVariant=Disabled  SumVariant=Sum_PID  TsampFilterVariant=InternalTs  TsampNgainVariant=Passthrough  TsampIntegralVariant=Disabled_SignalSpec  ExternalSaturationOutDataTypeStr=Inherit: Same as second input
  Out1 : Outport
  " " : Outport  Port=2
  wires:
  PID Controller (2DOF)/1 -> Display2/1, Out1/1
  [truepropEff] -> Display/1, PID Controller (2DOF)/2
  Reference/1 -> Display1/1, PID Controller (2DOF)/1
  States/1 -> " "/1

== system DA40_Flight_Model/Truth Model/Control/Subsystem5 ==
  Reference : Inport
  States : Inport  Port=2
  Out1 : Outport
  " " : Outport  Port=2
  wires:
  Reference/1 -> Out1/1
  States/1 -> " "/1

== system DA40_Flight_Model/Truth Model/Control/Subsystem6 ==
  Reference : Inport
  States : Inport  Port=2
  Out1 : Outport
  " " : Outport  Port=2
  wires:
  Reference/1 -> Out1/1
  States/1 -> " "/1

== system DA40_Flight_Model/Truth Model/Control/Subsystem7 ==
  Reference : Inport
  States : Inport  Port=2
  Out1 : Outport
  " " : Outport  Port=2
  wires:
  Reference/1 -> Out1/1
  States/1 -> " "/1

== system DA40_Flight_Model/Truth Model/Control/Subsystem8 ==
  Reference : Inport
  States : Inport  Port=2
  Out1 : Outport
  " " : Outport  Port=2
  wires:
  Reference/1 -> Out1/1
  States/1 -> " "/1

== system DA40_Flight_Model/Truth Model/Control/Subsystem9 ==
  Reference : Inport
  States : Inport  Port=2
  Out1 : Outport
  " " : Outport  Port=2
  wires:
  States/1 -> " "/1
  Reference/1 -> Out1/1
